simulink model "L4_3"  (R2023a)
settings: Solver=VariableStepAuto  StartTime=0.0  StopTime=7  RelTol=1e-8
undefined symbols (not defined in the file): k
settings Model: Creator=apere  LastModifiedBy=apere

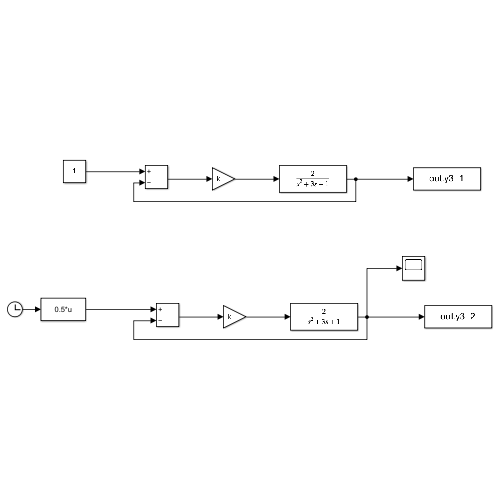
[thumbnail: Simulink's stored preview of the top-level diagram]
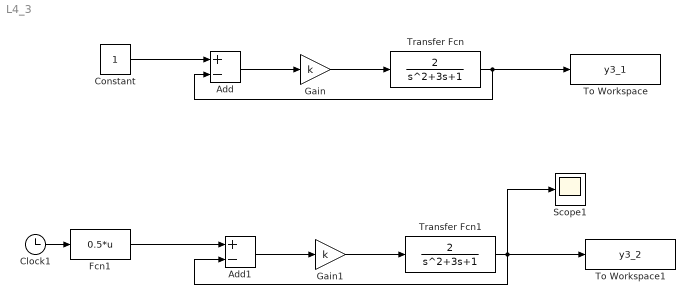
== system L4_3 ==
  Add : Sum  Inputs=+-
  Add1 : Sum  Inputs=+-
  Clock1 : Clock
  Constant : Constant
  Fcn1 : Fcn  Expr=0.5*u
  Gain : Gain  Gain=k
  Gain1 : Gain  Gain=k
  Scope1 : Scope
  To Workspace : ToWorkspace  VariableName=y3_1  SaveFormat=Timeseries  SampleTime=-1
  To Workspace1 : ToWorkspace  VariableName=y3_2  SaveFormat=Timeseries  SampleTime=-1
  Transfer Fcn : TransferFcn  Numerator=[2]  Denominator=[1 3 1]
  Transfer Fcn1 : TransferFcn  Numerator=[2]  Denominator=[1 3 1]
  wires:
  Gain/1 -> Transfer Fcn/1
  Add/1 -> Gain/1
  Transfer Fcn/1 -> To Workspace/1, Add/2
  Transfer Fcn1/1 -> To Workspace1/1, Add1/2, Scope1/1
  Fcn1/1 -> Add1/1
  Clock1/1 -> Fcn1/1
  Gain1/1 -> Transfer Fcn1/1
  Add1/1 -> Gain1/1
  Constant/1 -> Add/1
